simulink model "model_5LinkWalking"  (R2022b)
settings: Solver=ode45  StartTime=0.0  StopTime=Tf  FixedStep=1e-5  MaxStep=1e-3  RelTol=1e-12  AbsTol=1e-8
values from neighbouring files (symbols this model uses):
  f_dist = [0; -100; 0]    [main.m]    (also in main_5linkWalking_PSO.m)
  gains = [ ... (first row only)    [main.m]    (also in main_5linkWalking_PSO.m = [gain.kP1, gain.kD1, gain.kP2, gain.kD2, gain.kP3, gain.kD3,)
  gains_VSLIPSL = [gain_VSLIPSL.K_p; gain_VSLIPSL.K_d; gain_VSLIPSL.K_p_sw; gain_VSLIPSL.K_d_sw; gain_VSLIPSL.K_p_ds; gain_VSLIPSL.K_d_ds; gain_VSLIPSL.K_v_ds]    [main.m]    (also in main_5linkWalking_PSO.m)
  init_flag = [1; 0; -dc.col_param.footPlus; -slipsl.time_ss(N); slipsl.x_ss(1); slipsl.y_ss(1); alpha_ss_ref(1)]    [main.m]    (also in main_5linkWalking_PSO.m = [1; 0; -dc.col_param.footPlus; 0; CoM(1); CoM(2)])
  Initial_state = [q0;dq0]    [main.m]    (also in main_5linkWalking_PSO.m)
  param = [params.m1; params.m2; params.m5; params.l1; params.l2; params.l5; params.g; params.I1; params.I2; params.I5; params.r_k; params.r_h; params.k_ba; params.phi_h0; params.phi_k0]    [main.m]    (also in main_5linkWalking_PSO.m = [params.m1; params.m2; params.m5; params.l1; params.l2; para)
  ref_star_ds = [ref_star.ds.x_CoM_star,      ref_star.ds.y_CoM_star, ref_star.ds.dx_CoM_star,      ref_star.ds.del_y_CoM_star, ref_star.ds.del_dx_CoM_star,      ref_star.ds.del2_y_CoM_star]    [main.m]    (also in main_5linkWalking_PSO.m)
  ref_star_ss = [ref_star.ss.x_M_star,      ref_star.ss.y_M_star, ref_star.ss.x_swFoot_star, ref_star.ss.y_swFoot_star,      ref_star.ss.del_y_M_star, ref_star.ss.del_x_swFoot_star, ref_star.ss.del_y_swFoot_star,      ref_star.ss.del2_y_M_star, ref_star.ss.del2_x_swFoot_star, ref_star.ss.del2_y_swFoot_star,      ref_star.ss.x_CoM_star]    [main.m]    (also in main_5linkWalking_PSO.m)
  sample_time = 0.001    [main.m]    (also in main_5linkWalking_PSO.m)
  slipslParams = [ ... (first row only)    [main.m]    (also in main_5linkWalking_PSO.m)
  slipslTraj_ds = [slipsl.time_ds, slipsl.x_ds, slipsl.y_ds, slipsl.dx_ds, slipsl.dy_ds, alpha_ds_ref_discrete]    [main.m]    (also in main_5linkWalking_PSO.m = [ref_star.dc.ds.time - ref_star.dc.ds.time(1), ref_star.dc.d)
  slipslTraj_ss = [slipsl.time_ss, slipsl.x_ss, slipsl.y_ss, slipsl.dx_ss, slipsl.dy_ss, alpha_ss_ref_discrete]    [main.m]    (also in main_5linkWalking_PSO.m = [ref_star.dc.ss.time, ref_star.dc.ss.x_CoM', ref_star.dc.ss.)
  swFootTraj = [swFootSLIPSL.x_CoM, swFootSLIPSL.x, swFootSLIPSL.z, swFootSLIPSL.dx, swFootSLIPSL.dz]    [main.m]    (also in main_5linkWalking_PSO.m = [ref_star.dc.ss.x_CoM', ref_star.dc.ss.x_sw', ref_star.dc.ss)
libraries: simulink x1
(part 1 of 3)
settings Model: Creator=yamakita_lab  LastModifiedBy=mmpel
settings SolverCC: AutoScaleAbsTol=off  AlgebraicLoopSolver=TrustRegion
settings DataIOCC: ReturnWorkspaceOutputs=off
settings DebuggingCC: UnconnectedInputMsg=warning  UnconnectedOutputMsg=warning  UnconnectedLineMsg=warning  SFMachineParentedDataDiag=warning  ArithmeticOperatorsInVariantConditions=warning
settings ModelReferenceCC: EnableRefExpFcnMdlSchedulingChecks=on
settings SFSimCC: SimUseLocalCustomCode=off  CustomCodeUndefinedFunction=UseInterfaceOnly
settings RTWCC: RTWUseLocalCustomCode=off  DLArmComputeVersion=19.05

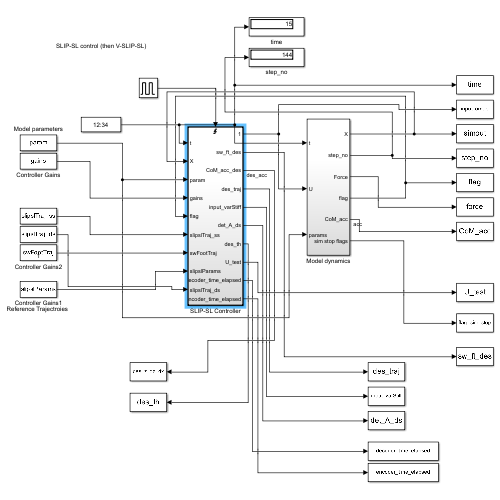
[thumbnail: Simulink's stored preview of the top-level diagram]
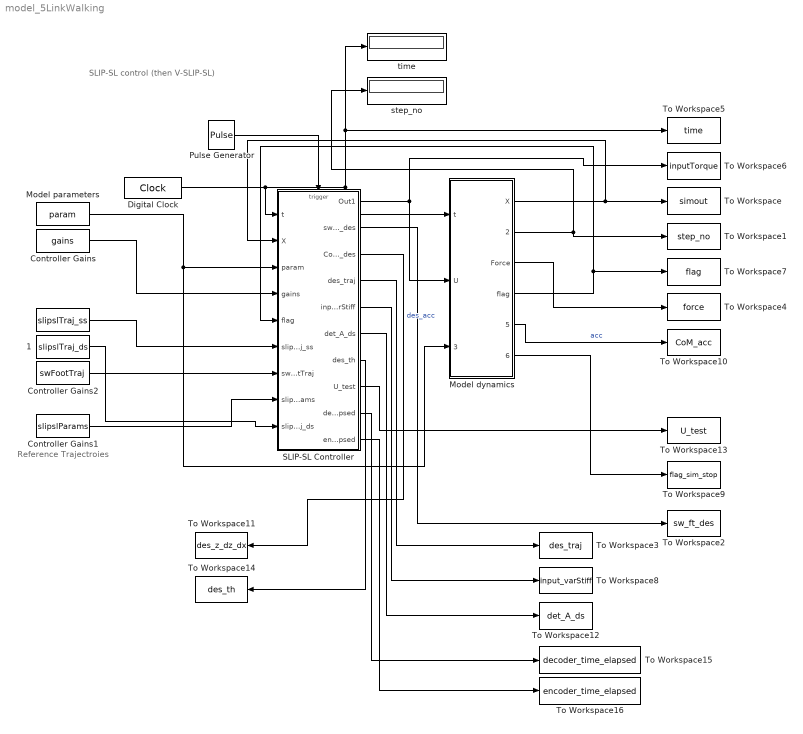
== system model_5LinkWalking ==
  note: Reference Trajectroies
  note: SLIP-SL control (then V-SLIP-SL)
  " " : Constant  Value=slipslTraj_ss
  " 1" : Constant  Value=slipslTraj_ds
  Controller Gains : Constant  Value=gains
  Controller Gains1 : Constant  Value=slipslParams
  Controller Gains2 : Constant  Value=swFootTraj
  Digital Clock : DigitalClock  SampleTime=1e-4
  Model dynamics : Subsystem
  Model parameters : Constant  Value=param  OutDataTypeStr=double
  Pulse Generator : DiscretePulseGenerator  PulseType=Time based  Period=5e-4  PulseWidth=5
  SLIP-SL Controller : Subsystem  TreatAsAtomicUnit=on
  To Workspace : ToWorkspace  VariableName=simout  SampleTime=sample_time
  To Workspace1 : ToWorkspace  VariableName=step_no  SampleTime=sample_time
  To Workspace10 : ToWorkspace  VariableName=CoM_acc  SampleTime=sample_time
  To Workspace11 : ToWorkspace  VariableName=des_z_dz_dx  SampleTime=sample_time
  To Workspace12 : ToWorkspace  VariableName=det_A_ds  SampleTime=sample_time
  To Workspace13 : ToWorkspace  VariableName=U_test  SampleTime=sample_time
  To Workspace14 : ToWorkspace  VariableName=des_th  SampleTime=sample_time
  To Workspace15 : ToWorkspace  VariableName=decoder_time_elapsed  SampleTime=sample_time
  To Workspace16 : ToWorkspace  VariableName=encoder_time_elapsed  SampleTime=sample_time
  To Workspace2 : ToWorkspace  VariableName=sw_ft_des  SampleTime=sample_time
  To Workspace3 : ToWorkspace  VariableName=des_traj  SampleTime=sample_time
  To Workspace4 : ToWorkspace  VariableName=force  SampleTime=sample_time
  To Workspace5 : ToWorkspace  VariableName=time  SampleTime=sample_time
  To Workspace6 : ToWorkspace  VariableName=inputTorque  SampleTime=sample_time
  To Workspace7 : ToWorkspace  VariableName=flag  SampleTime=sample_time
  To Workspace8 : ToWorkspace  VariableName=input_varStiff  SampleTime=sample_time
  To Workspace9 : ToWorkspace  VariableName=flag_sim_stop  SampleTime=sample_time
  step_no : Display
  time : Display
  wires:
  SLIP-SL Controller/1(Out1) -> Model dynamics/2(U), To Workspace6/1
  Model dynamics/1(X) -> SLIP-SL Controller/2(X), To Workspace/1
  Digital Clock/1 -> SLIP-SL Controller/1(t), time/1, To Workspace5/1, Model dynamics/1(t)
  Model dynamics/2(step_no) -> step_no/1, To Workspace1/1
  SLIP-SL Controller/2(sw_ft_des) -> To Workspace2/1
  Model dynamics/3(Force) -> To Workspace4/1
  Model parameters/1 -> Model dynamics/3(params), SLIP-SL Controller/3(param)
  Controller Gains/1 -> SLIP-SL Controller/4(gains)
  Model dynamics/4(flag) -> To Workspace7/1, SLIP-SL Controller/5(flag)
  SLIP-SL Controller/3(CoM_acc_des) -> To Workspace11/1  "des_acc"
  Model dynamics/5(CoM_acc) -> To Workspace10/1  "acc"
  " "/1 -> SLIP-SL Controller/6(slipslTraj_ss)
  Controller Gains2/1 -> SLIP-SL Controller/7(swFootTraj)
  Pulse Generator/1 -> SLIP-SL Controller/Trigger
  Model dynamics/6(sim stop flags) -> To Workspace9/1
  Controller Gains1/1 -> SLIP-SL Controller/8(slipslParams)
  SLIP-SL Controller/4(des_traj) -> To Workspace3/1
  SLIP-SL Controller/5(input_varStiff) -> To Workspace8/1
  SLIP-SL Controller/6(det_A_ds) -> To Workspace12/1
  SLIP-SL Controller/7(des_th) -> To Workspace14/1
  " 1"/1 -> SLIP-SL Controller/9(slipslTraj_ds)
  SLIP-SL Controller/8(U_test) -> To Workspace13/1
  SLIP-SL Controller/9(decoder_time_elapsed) -> To Workspace15/1
  SLIP-SL Controller/10(encoder_time_elapsed) -> To Workspace16/1

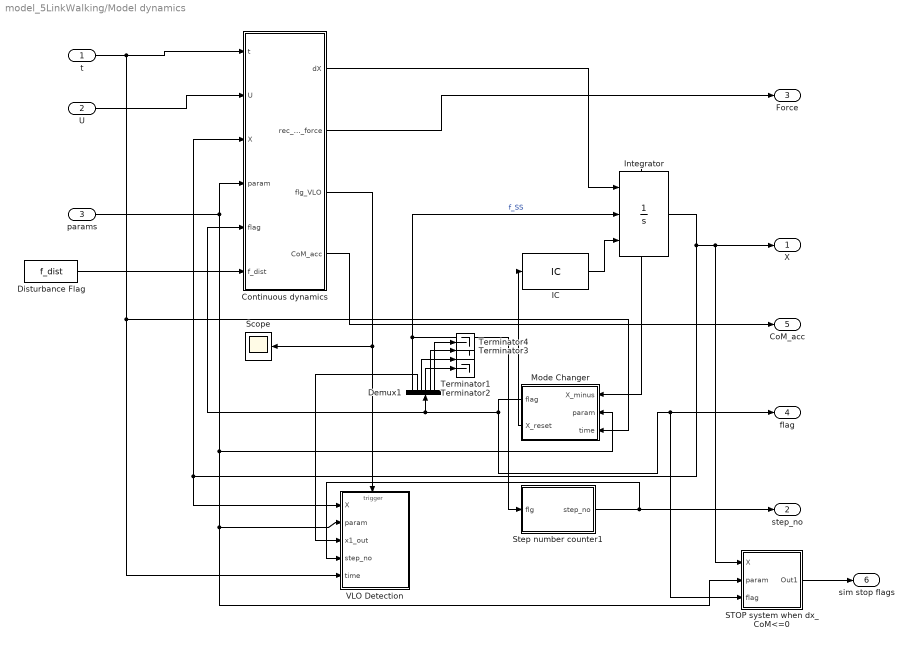
== system model_5LinkWalking/Model dynamics ==
  t : Inport
  U : Inport  Port=2
  params : Inport  Port=3
  Continuous dynamics : MATLAB Function  TreatAsAtomicUnit=on
  Demux1 : Demux  Outputs=6
  Disturbance Flag : Constant  Value=f_dist
  IC : InitialCondition  Value=Initial_state
  Integrator : Integrator  ExternalReset=falling  InitialConditionSource=external  ShowStatePort=on
  Mode Changer : Subsystem
  STOP system when dx_CoM<=0 : Subsystem
  Scope : Scope
  Step number counter1 : Subsystem
  Terminator{1..4} (4 alike) : Terminator
  VLO Detection : Subsystem  TreatAsAtomicUnit=on
  X : Outport  VectorParamsAs1DForOutWhenUnconnected=off
  step_no : Outport  Port=2  VectorParamsAs1DForOutWhenUnconnected=off
  Force : Outport  Port=3  VectorParamsAs1DForOutWhenUnconnected=off
  flag : Outport  Port=4
  CoM_acc : Outport  Port=5  VectorParamsAs1DForOutWhenUnconnected=off
  sim stop flags : Outport  Port=6
  wires:
  IC/1 -> Integrator/3
  Integrator/State -> Mode Changer/1(X_minus)
  Continuous dynamics/1(dX) -> Integrator/1
  params/1 -> Continuous dynamics/4(param), STOP system when dx_CoM<=0/2(param), VLO Detection/2(param), Mode Changer/2("param ")
  U/1 -> Continuous dynamics/2(U)
  t/1 -> Continuous dynamics/1(t), VLO Detection/5(time), Mode Changer/3(time)
  Continuous dynamics/3(flg_VLO) -> Scope/1, VLO Detection/Trigger
  Integrator/1 -> STOP system when dx_CoM<=0/1(X), X/1, Continuous dynamics/3(X), VLO Detection/1(X)
  Mode Changer/2(X_reset) -> IC/1
  Mode Changer/1(flag) -> STOP system when dx_CoM<=0/3(flag), flag/1, Demux1/1, Continuous dynamics/5(flag)
  Demux1/2 -> VLO Detection/3(x1_out)
  Demux1/3 -> Terminator1/1
  Demux1/1 -> Step number counter1/1(flg), Integrator/2  "f_SS"
  Step number counter1/1(step_no) -> VLO Detection/4(step_no), step_no/1
  Continuous dynamics/4(CoM_acc) -> CoM_acc/1
  Continuous dynamics/2(rec_cs_force) -> Force/1
  Demux1/4 -> Terminator2/1
  Demux1/5 -> Terminator3/1
  Demux1/6 -> Terminator4/1
  STOP system when dx_CoM<=0/1(Out1) -> sim stop flags/1
  Disturbance Flag/1 -> Continuous dynamics/6(f_dist)

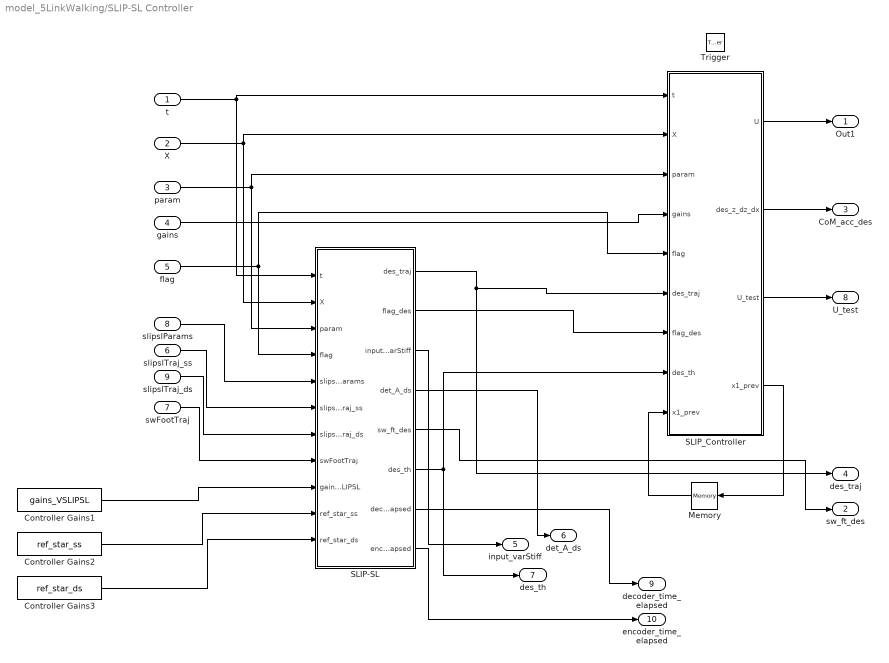
== system model_5LinkWalking/SLIP-SL Controller ==
  t : Inport
  X : Inport  Port=2
  param : Inport  Port=3
  gains : Inport  Port=4
  flag : Inport  Port=5
  slipslTraj_ss : Inport  Port=6
  swFootTraj : Inport  Port=7
  slipslParams : Inport  Port=8
  slipslTraj_ds : Inport  Port=9
  Trigger : TriggerPort  VariantControl=Variant  PortDimensions=1
  Controller Gains1 : Constant  Value=gains_VSLIPSL
  Controller Gains2 : Constant  Value=ref_star_ss
  Controller Gains3 : Constant  Value=ref_star_ds
  Memory : Memory  InitialCondition=[0, 0]  InheritSampleTime=on
  SLIP-SL : MATLAB Function  TreatAsAtomicUnit=on
  SLIP_Controller : MATLAB Function  TreatAsAtomicUnit=on
  Out1 : Outport  VectorParamsAs1DForOutWhenUnconnected=off
  sw_ft_des : Outport  Port=2  VectorParamsAs1DForOutWhenUnconnected=off
  CoM_acc_des : Outport  Port=3  VectorParamsAs1DForOutWhenUnconnected=off
  des_traj : Outport  Port=4  VectorParamsAs1DForOutWhenUnconnected=off
  input_varStiff : Outport  Port=5  VectorParamsAs1DForOutWhenUnconnected=off
  det_A_ds : Outport  Port=6  VectorParamsAs1DForOutWhenUnconnected=off
  des_th : Outport  Port=7  VectorParamsAs1DForOutWhenUnconnected=off
  U_test : Outport  Port=8  VectorParamsAs1DForOutWhenUnconnected=off
  decoder_time_elapsed : Outport  Port=9  VectorParamsAs1DForOutWhenUnconnected=off
  encoder_time_elapsed : Outport  Port=10  VectorParamsAs1DForOutWhenUnconnected=off
  wires:
  SLIP_Controller/1(U) -> Out1/1
  t/1 -> SLIP-SL/1(t), SLIP_Controller/1(t)
  X/1 -> SLIP-SL/2(X), SLIP_Controller/2(X)
  param/1 -> SLIP_Controller/3(param), SLIP-SL/3(param)
  SLIP-SL/5(sw_ft_des) -> sw_ft_des/1
  Memory/1 -> SLIP_Controller/9("x1_prev ")
  SLIP_Controller/4(x1_prev) -> Memory/1
  gains/1 -> SLIP_Controller/4(gains)
  flag/1 -> SLIP_Controller/5(flag), SLIP-SL/4(flag)
  SLIP_Controller/2(des_z_dz_dx) -> CoM_acc_des/1
  slipslTraj_ss/1 -> SLIP-SL/6(slipslTraj_ss)
  swFootTraj/1 -> SLIP-SL/8(swFootTraj)
  SLIP-SL/1(des_traj) -> des_traj/1, SLIP_Controller/6(des_traj)
  SLIP-SL/2(flag_des) -> SLIP_Controller/7(flag_des)
  slipslParams/1 -> SLIP-SL/5(slipslParams)
  Controller Gains1/1 -> SLIP-SL/9(gains_VSLIPSL)
  Controller Gains2/1 -> SLIP-SL/10(ref_star_ss)
  Controller Gains3/1 -> SLIP-SL/11(ref_star_ds)
  SLIP-SL/3(input_varStiff) -> input_varStiff/1
  SLIP-SL/4(det_A_ds) -> det_A_ds/1
  SLIP-SL/6(des_th) -> des_th/1, SLIP_Controller/8(des_th)
  slipslTraj_ds/1 -> SLIP-SL/7(slipslTraj_ds)
  SLIP_Controller/3(U_test) -> U_test/1
  SLIP-SL/7(decoder_time_elapsed) -> decoder_time_elapsed/1
  SLIP-SL/8(encoder_time_elapsed) -> encoder_time_elapsed/1

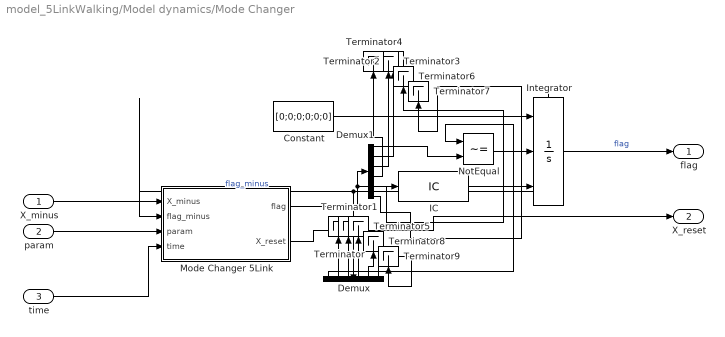
== system model_5LinkWalking/Model dynamics/Mode Changer ==
  X_minus : Inport
  "param " : Inport  Port=2
  time : Inport  Port=3
  Constant : Constant  Value=[0;0;0;0;0;0]
  Demux : Demux  Outputs=6
  Demux1 : Demux  Outputs=6
  IC : InitialCondition  Value=init_flag
  Integrator : Integrator  ExternalReset=rising  InitialConditionSource=external  ShowStatePort=on
  Mode Changer 5Link : MATLAB Function  TreatAsAtomicUnit=on
  NotEqual : RelationalOperator  Operator=~=  OutDataTypeStr=boolean  RndMeth=Simplest  InputSameDT=off
  Terminator{,1..9} (10 alike) : Terminator
  flag : Outport  VectorParamsAs1DForOutWhenUnconnected=off
  X_reset : Outport  Port=2  VectorParamsAs1DForOutWhenUnconnected=off
  wires:
  X_minus/1 -> Mode Changer 5Link/1(X_minus)
  IC/1 -> Integrator/3
  Integrator/State -> Mode Changer 5Link/2(flag_minus), Demux/1  "flag_minus"
  "param "/1 -> Mode Changer 5Link/3(param)
  Mode Changer 5Link/1(flag) -> Demux1/1, IC/1
  Constant/1 -> Integrator/1
  NotEqual/1 -> Integrator/2
  Integrator/1 -> flag/1  "flag"
  Mode Changer 5Link/2(X_reset) -> X_reset/1
  Demux/1 -> NotEqual/1
  Demux/3 -> Terminator1/1
  Demux/2 -> Terminator/1
  Demux1/1 -> NotEqual/2
  Demux1/2 -> Terminator2/1
  Demux1/3 -> Terminator3/1
  time/1 -> Mode Changer 5Link/4(time)
  Demux1/4 -> Terminator4/1
  Demux/4 -> Terminator5/1
  Demux/5 -> Terminator8/1
  Demux/6 -> Terminator9/1
  Demux1/5 -> Terminator6/1
  Demux1/6 -> Terminator7/1

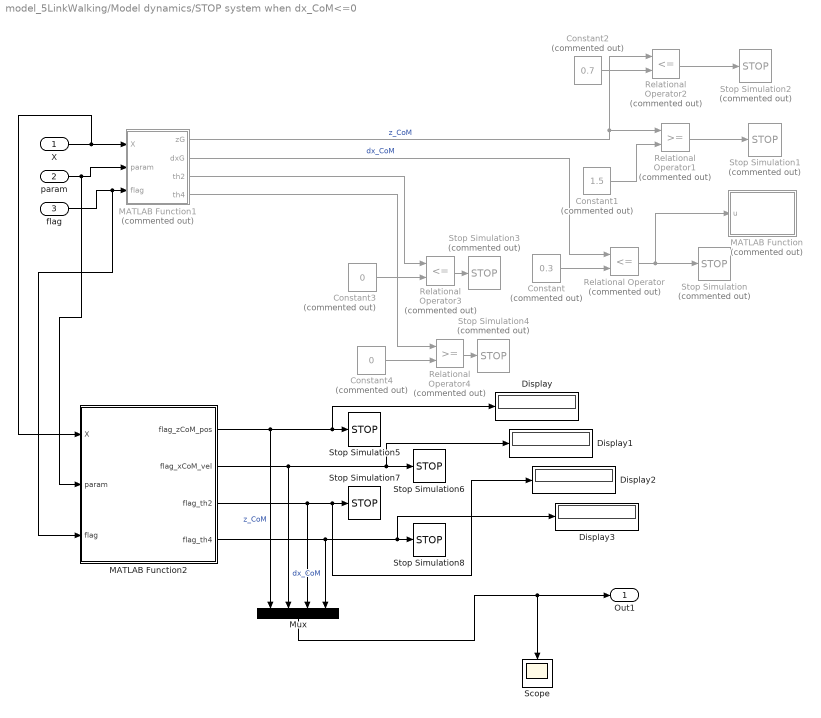
== system model_5LinkWalking/Model dynamics/STOP system when dx_CoM<=0 ==
  X : Inport
  param : Inport  Port=2
  flag : Inport  Port=3
  Constant : Constant  Commented=on  Value=0.3
  Constant1 : Constant  Commented=on  Value=1.5
  Constant2 : Constant  Commented=on  Value=0.7
  Constant3 : Constant  Commented=on  Value=0
  Constant4 : Constant  Commented=on  Value=0
  Display{,1..3} (4 alike) : Display
  MATLAB Function : MATLAB Function  Commented=on  TreatAsAtomicUnit=on
  MATLAB Function1 : MATLAB Function  Commented=on  TreatAsAtomicUnit=on
  MATLAB Function2 : MATLAB Function  TreatAsAtomicUnit=on
  Mux : Mux
  Relational Operator : RelationalOperator  Commented=on  Operator=<=  OutDataTypeStr=boolean  RndMeth=Simplest  InputSameDT=off
  Relational Operator1 : RelationalOperator  Commented=on  OutDataTypeStr=boolean  RndMeth=Simplest  InputSameDT=off
  Relational Operator2 : RelationalOperator  Commented=on  Operator=<=  OutDataTypeStr=boolean  RndMeth=Simplest  InputSameDT=off
  Relational Operator3 : RelationalOperator  Commented=on  Operator=<=  OutDataTypeStr=boolean  RndMeth=Simplest  InputSameDT=off
  Relational Operator4 : RelationalOperator  Commented=on  OutDataTypeStr=boolean  RndMeth=Simplest  InputSameDT=off
  Scope : Scope
  Stop Simulation{,1..4} (5 alike) : Stop  Commented=on
  Stop Simulation{5..8} (4 alike) : Stop
  Out1 : Outport
  wires:
  Constant/1 -> Relational Operator/2
  Relational Operator/1 -> Stop Simulation/1, MATLAB Function/1(u)
  MATLAB Function1/2(dxG) -> Relational Operator/1  "dx_CoM"
  MATLAB Function1/1(zG) -> Relational Operator2/1, Relational Operator1/1  "z_CoM"
  Relational Operator1/1 -> Stop Simulation1/1
  Constant1/1 -> Relational Operator1/2
  Relational Operator2/1 -> Stop Simulation2/1
  Constant2/1 -> Relational Operator2/2
  X/1 -> MATLAB Function2/1(X), MATLAB Function1/1(X)
  param/1 -> MATLAB Function2/2(param), MATLAB Function1/2(param)
  flag/1 -> MATLAB Function2/3(flag), MATLAB Function1/3(flag)
  MATLAB Function1/3(th2) -> Relational Operator3/1
  Constant3/1 -> Relational Operator3/2
  MATLAB Function1/4(th4) -> Relational Operator4/1
  Constant4/1 -> Relational Operator4/2
  Relational Operator3/1 -> Stop Simulation3/1
  Relational Operator4/1 -> Stop Simulation4/1
  MATLAB Function2/1(flag_zCoM_pos) -> Mux/1, Display/1, Stop Simulation5/1  "z_CoM"
  MATLAB Function2/2(flag_xCoM_vel) -> Mux/2, Display1/1, Stop Simulation6/1  "dx_CoM"
  MATLAB Function2/3(flag_th2) -> Display2/1, Stop Simulation7/1, Mux/3
  MATLAB Function2/4(flag_th4) -> Mux/4, Display3/1, Stop Simulation8/1
  Mux/1 -> Scope/1, Out1/1

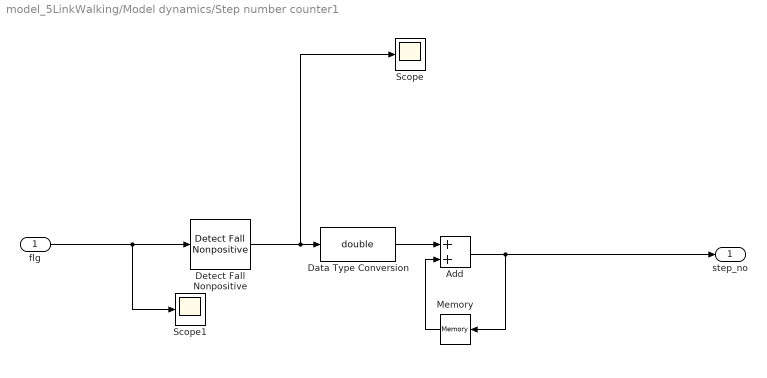
== system model_5LinkWalking/Model dynamics/Step number counter1 ==
  flg : Inport  SampleTime=sample_time
  Add : Sum
  Data Type Conversion : DataTypeConversion  OutDataTypeStr=double  SaturateOnIntegerOverflow=off  RndMeth=Floor
  Detect Fall Nonpositive : simulink/Logic and Bit Operations/Detect Fall Nonpositive  vinit=1  OutDataTypeStr=boolean
  Memory : Memory  InheritSampleTime=on
  Scope : Scope
  Scope1 : Scope
  step_no : Outport  VectorParamsAs1DForOutWhenUnconnected=off
  wires:
  Add/1 -> step_no/1, Memory/1
  Memory/1 -> Add/2
  Detect Fall Nonpositive/1 -> Scope/1, Data Type Conversion/1
  flg/1 -> Detect Fall Nonpositive/1, Scope1/1
  Data Type Conversion/1 -> Add/1

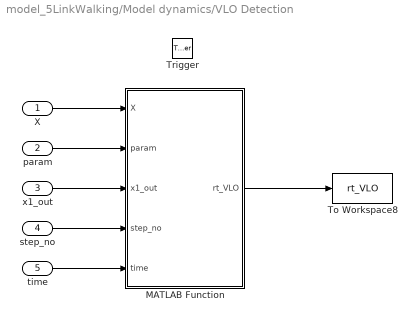
== system model_5LinkWalking/Model dynamics/VLO Detection ==
  X : Inport
  param : Inport  Port=2
  x1_out : Inport  Port=3
  step_no : Inport  Port=4
  time : Inport  Port=5
  Trigger : TriggerPort  VariantControl=Variant
  MATLAB Function : MATLAB Function  TreatAsAtomicUnit=on
  To Workspace8 : ToWorkspace  VariableName=rt_VLO  SampleTime=-1
  wires:
  X/1 -> MATLAB Function/1(X)
  MATLAB Function/1(rt_VLO) -> To Workspace8/1
  param/1 -> MATLAB Function/2(param)
  x1_out/1 -> MATLAB Function/3(x1_out)
  step_no/1 -> MATLAB Function/4(step_no)
  time/1 -> MATLAB Function/5(time)

== matlab function model_5LinkWalking/Model dynamics/VLO Detection/MATLAB Function ==
  data: X input; rt_VLO output; param input; x1_out input; step_no input; time input
function rt_VLO = fcn(X, param, x1_out, step_no, time)

CoM = calculate_com(X, param, x1_out, [0;0;0;0;0]); % calculation the CoM location

z_CoM = CoM(2);
dx_CoM = CoM(3);
dz_CoM = CoM(4);
theta_P = atan2(dz_CoM, dx_CoM);
z_P = z_CoM;

total_CoM_E = calculate_CoM_energy(X, param); % total energy of CoM @VLO
% total_E = calculate_total_energy(X, param); % total energy of robot @VLO

rt_VLO =[theta_P, z_P, step_no, total_CoM_E, time];

== matlab function model_5LinkWalking/Model dynamics/Mode Changer/Mode Changer 5Link ==
  data: X_minus input; flag output; flag_minus input; param input; X_reset output; time input
function [flag, X_reset]  = fcn(X_minus, flag_minus, param, time)

%% variables

th1 = X_minus(1);
th2 = X_minus(2);
th3 = X_minus(3);
th4 = X_minus(4);
th5 = X_minus(5);

dth1 = X_minus(6);
dth2 = X_minus(7);
dth3 = X_minus(8);
dth4 = X_minus(9);
dth5 = X_minus(10);

q = [th1;th2;th3;th4;th5];
dq = [dth1;dth2;dth3;dth4;dth5];

%% parameters

m1 = param(1);
m2 = param(2);
m3 = m2;
m4 = m1;
m5 = param(3);

l1 = param(4);
l2 = param(5);
l5 = param(6);
l3 = l2;
l4 = l1;

gravi = param(7);
I1 = param(8);
I2 = param(9);
I5 = param(10);
I3 = I1;
I4 = I2;

q_minus = [th1;th2;th3;th4;th5];
dq_minus = [dth1;dth2;dth3;dth4;dth5];

%% flags
f_SS = flag_minus(1); % indicates which stance phase it is
foot = flag_minus(2); % location of the stance foot
foot_prev = flag_minus(3); % previous location of the stance foot
% time = flag_minus(4); % previous location of the stance foot
x_LO = flag_minus(5); % x_CoM location when liftOff happens
z_LO = flag_minus(6); % z_CoM location when liftOff happens

%%
X_reset = [q_minus; dq_minus]; % dummy X_reset so that simulink doesn't give error

%% calculating the Swing foot position and velocity
Psw_tip_minus = [l1*cos(th1) + l2*cos(th1 + th2) + l3*cos(th1 + th2 + th3) + l4*cos(th1 + th2 + th3 + th4);
                 l1*sin(th1) + l2*sin(th1 + th2) + l3*sin(th1 + th2 + th3) + l4*sin(th1 + th2 + th3 + th4)];
 
J_Psw_tip_minus = [- l4*sin(th1 + th2 + th3 + th4) - l2*sin(th1 + th2) - l1*sin(th1) - l3*sin(th1 + th2 + th3), - l4*sin(th1 + th2 + th3 + th4) - l2*sin(th1 + th2) - l3*sin(th1 + th2 + th3), - l4*sin(th1 + th2 + th3 + th4) - l3*sin(th1 + th2 + th3), -l4*sin(th1 + th2 + th3 + th4), 0;
                   l4*cos(th1 + th2 + th3 + th4) + l2*cos(th1 + th2) + l1*cos(th1) + l3*cos(th1 + th2 + th3),   l4*cos(th1 + th2 + th3 + th4) + l2*cos(th1 + th2) + l3*cos(th1 + th2 + th3),   l4*cos(th1 + th2 + th3 + th4) + l3*cos(th1 + th2 + th3),  l4*cos(th1 + th2 + th3 + th4), 0];

dPsw_tip_minus = J_Psw_tip_minus*dq_minus;

% debugging
if time > 6
    step_distance = 0;
end

%%
step_distance = 0;

% % if f_SS == 1 && Psw_tip_minus(2,1) <= 0.005 && dPsw_tip_minus(2,1) < -0.5
% if f_SS == 1 && Psw_tip_minus(2,1) <= 0 && dPsw_tip_minus(2,1) < -0.01
%     % change from single stance phase to double stance phase
%     f_SS = -1;
%     foot_prev = foot; % saving the old foot location
%     foot = foot_prev + Psw_tip_minus(1,1); % calculating the new foots location
%            
%     % Impact mapによる衝突後の状態の計算
%     MM_minus = MM_matrix(X_minus,param);
%     dq_after = (eye(5)-inv(MM_minus)*J_Psw_tip_minus'*inv(J_Psw_tip_minus*inv(MM_minus)*J_Psw_tip_minus')*J_Psw_tip_minus)*dq_minus;
%     
%     th1_after = q_minus(4,1) + q_minus(3,1) + q_minus(2,1) + q_minus(1,1) - pi; % th1 becomes th4
%     th2_after = - q_minus(4,1); % th2 becomes th3
%     th3_after = - q_minus(3,1); % th3 becomes th2
%     th4_after = - q_minus(2,1); % th4 becomes th1
%     th5_after = q_minus(5,1) - q_minus(3,1) + pi;
%     
%     q_after = [th1_after; th2_after; th3_after; th4_after; th5_after]; % this is where the switching happens
%     
%     dth1_after = dq_after(4,1) + dq_after(3,1) + dq_after(2,1) + dq_after(1,1); % th1 becomes th4
%     dth2_after = - dq_after(4,1); % th2 becomes th3
%     dth3_after = - dq_after(3,1); % th3 becomes th2
%     dth4_after = - dq_after(2,1); % th4 becomes th1
%     dth5_after = dq_after(5,1) - dq_after(3,1);
%     
%     % recording step location because system model in non-floating base
%     step_distance = Psw_tip_minus(1,1);
%     
%     % Reset state if the f_ss change from 1 to 0 (from single stance to
%     % double stance)
%     X_reset = [q_after; dth1_after; dth2_after; dth3_after; dth4_after; dth5_after];
% 
% % elseif f_SS == -1 && constraint_force(2) < 0
% % elseif f_SS == -1 && dPsw_tip_minus(2,1) > 0.005

if f_SS == 1 && Psw_tip_minus(2,1) <= 0 && ( ( Psw_tip_minus(1,1) > 0 && dPsw_tip_minus(2,1) <= 0) || ( Psw_tip_minus(1,1) <= 0 && dPsw_tip_minus(2,1) <= -0.5) )
    % change from single stance phase to double stance phase
    f_SS = -1;
    foot_prev = foot; % saving the old foot location
    foot = foot_prev + Psw_tip_minus(1,1); % calculating the new foots location
           
    % Impact mapによる衝突後の状態の計算
    MM_minus = MM_matrix(X_minus,param);
    dq_after = (eye(5)-inv(MM_minus)*J_Psw_tip_minus'*inv(J_Psw_tip_minus*inv(MM_minus)*J_Psw_tip_minus')*J_Psw_tip_minus)*dq_minus;
    
    th1_after = q_minus(4,1) + q_minus(3,1) + q_minus(2,1) + q_minus(1,1) - pi; % th1 becomes th4
    th2_after = - q_minus(4,1); % th2 becomes th3
    th3_after = - q_minus(3,1); % th3 becomes th2
    th4_after = - q_minus(2,1); % th4 becomes th1
    th5_after = q_minus(5,1) - q_minus(3,1) + pi;
    
    q_after = [th1_after; th2_after; th3_after; th4_after; th5_after]; % this is where the switching happens
    
    dth1_after = dq_after(4,1) + dq_after(3,1) + dq_after(2,1) + dq_after(1,1); % th1 becomes th4
    dth2_after = - dq_after(4,1); % th2 becomes th3
    dth3_after = - dq_after(3,1); % th3 becomes th2
    dth4_after = - dq_after(2,1); % th4 becomes th1
    dth5_after = dq_after(5,1) - dq_after(3,1);
    
    % recording step location because system model in non-floating base
    step_distance = Psw_tip_minus(1,1);
    
    % Reset state if the f_ss change from 1 to 0 (from single stance to
    % double stance)
    X_reset = [q_after; dth1_after; dth2_after; dth3_after; dth4_after; dth5_after];

% elseif f_SS == -1 && constraint_force(2) < 0
% elseif f_SS == -1 && dPsw_tip_minus(2,1) > 0.005
elseif f_SS == -1 && dPsw_tip_minus(2,1) > 0.005
% elseif f_SS == -1 && abs(dPsw_tip_minus(2,1)) > 1e-5
    % change from double stance phase to single stance phase if the y
    % component of the contraint force becomes negative
    f_SS = 1;
    % reset X to restart swing leg with zero initial velocity from the
    % position that swing leg last was
    X_reset = X_minus;
    
    % calculating CoM pos
    CoM = calculate_com(X_minus, param, foot, [0;0;0;0;0]);
    x_LO = CoM(1);
    z_LO = CoM(2);        
end

flag = [f_SS; foot; foot_prev; time; x_LO; z_LO];

== matlab function model_5LinkWalking/Model dynamics/STOP system when dx_CoM<=0/MATLAB Function2 ==
  data: X input; param input; flag input; flag_zCoM_pos output; flag_xCoM_vel output; flag_th2 output; flag_th4 output
function [flag_zCoM_pos, flag_xCoM_vel, flag_th2, flag_th4] = fcn(X,param, flag)

%% variables
th1 = X(1);
th2 = X(2);
th3 = X(3);
th4 = X(4);
th5 = X(5);

dth1 = X(6);
dth2 = X(7);
dth3 = X(8);
dth4 = X(9);
dth5 = X(10);

q = [th1;th2;th3;th4;th5];
dq = [dth1;dth2;dth3;dth4;dth5];

%% parameters

m1 = param(1);
m2 = param(2);
m3 = m2;
m4 = m1;
m5 = param(3);

l1 = param(4);
l2 = param(5);
l5 = param(6);
l3 = l2;
l4 = l1;

gravi = param(7);
I1 = param(8);
I2 = param(9);
I5 = param(10);
I3 = I1;
I4 = I2;

%% flags
f_SS = flag(1); % indicates which stance phase it is
foot = flag(2); % location of the stance foot
foot_prev = flag(3); % previous location of the stance foot

%% CoM calculation
% CoM = [xG, zG, dxG, dzG, ddxG, ddzG];
CoM = calculate_com(X, param, 0, [0;0;0;0;0]); % calculation the CoM location

xG = CoM(1);
zG = CoM(2);
dxG = CoM(3);
dzG = CoM(4);

%%

% flag_zCoM_pos: if z_CoM drops or rises above certain value
flag_zCoM_pos = 0;
if zG >= 1.5
    flag_zCoM_pos = 1;
elseif zG <= 0.7
    flag_zCoM_pos = 1;
end

% flag_xCoM_vel
flag_xCoM_vel = 0;
% if dxG <= 0
%     flag_xCoM_vel = 1;
% end

% flag_th2
flag_th2 = 0;
if mod(th2, 2*pi) <= 0
    flag_th2 = 1;
end

% flag_th4
flag_th4 = 0;
if th4 >= 0
%     flag_th4 = 1;
end
